simulink model "DynamicModel_Cascaded_BAv02"  (R2022b)
settings: Solver=VariableStepAuto  StartTime=0.0  StopTime=9*3600  MaxStep=0.2  RelTol=1e-3
undefined symbols (not defined in the file): driver, getPhysicalConstants, param, route, weatherSim
libraries: slpidlib x4
settings Model: NumberOfSteps=100  Creator=giaco  LastModifiedBy=giaco

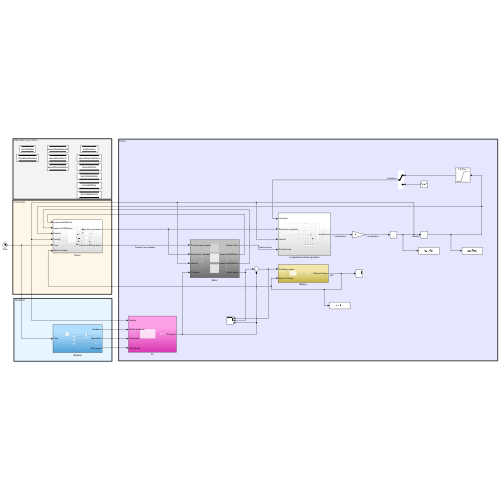
[thumbnail: Simulink's stored preview of the top-level diagram]
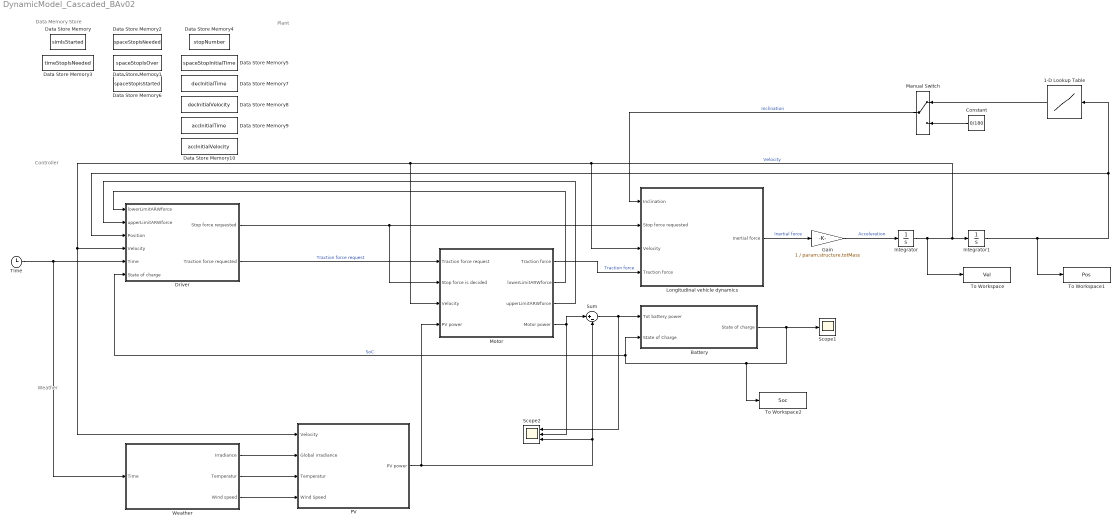
== system DynamicModel_Cascaded_BAv02 ==
  note: Weather
  note: Controller
  note: Plant
  note: Data Memory Store
  1-D Lookup Table : Lookup_n-D  NumberOfTableDimensions=1  BreakpointsForDimension1=route.dist(1:end-1)  Table=route.inclSmooth  InternalRulePriority=Speed  RndMeth=Simplest
  Battery : Subsystem
  Constant : Constant  Value=0/180
  Data Store Memory : DataStoreMemory  DataStoreName=simIsStarted  WriteAfterWriteMsg=warning  InitialValue=true  ShowAdditionalParam=off  OutDataTypeStr=boolean
  Data Store Memory1 : DataStoreMemory  DataStoreName=spaceStopIsOver  WriteAfterWriteMsg=warning  InitialValue=false  ShowAdditionalParam=off  OutDataTypeStr=boolean
  Data Store Memory10 : DataStoreMemory  DataStoreName=accInitialVelocity  WriteAfterWriteMsg=warning  VectorParams1D=off  ShowAdditionalParam=off  OutDataTypeStr=double
  Data Store Memory2 : DataStoreMemory  DataStoreName=spaceStopIsNeeded  WriteAfterWriteMsg=warning  InitialValue=false  ShowAdditionalParam=off  OutDataTypeStr=boolean
  Data Store Memory3 : DataStoreMemory  DataStoreName=timeStopIsNeeded  WriteAfterWriteMsg=warning  InitialValue=false  ShowAdditionalParam=off  OutDataTypeStr=boolean
  Data Store Memory4 : DataStoreMemory  DataStoreName=stopNumber  WriteAfterWriteMsg=warning  InitialValue=2  VectorParams1D=off  ShowAdditionalParam=off  OutDataTypeStr=int8
  Data Store Memory5 : DataStoreMemory  DataStoreName=spaceStopInitialTime  WriteAfterWriteMsg=warning  VectorParams1D=off  ShowAdditionalParam=off  OutDataTypeStr=double
  Data Store Memory6 : DataStoreMemory  DataStoreName=spaceStopIsStarted  WriteAfterWriteMsg=warning  InitialValue=false  ShowAdditionalParam=off  OutDataTypeStr=boolean
  Data Store Memory7 : DataStoreMemory  DataStoreName=decInitialTime  WriteAfterWriteMsg=warning  VectorParams1D=off  ShowAdditionalParam=off  OutDataTypeStr=double
  Data Store Memory8 : DataStoreMemory  DataStoreName=decInitialVelocity  WriteAfterWriteMsg=warning  VectorParams1D=off  ShowAdditionalParam=off  OutDataTypeStr=double
  Data Store Memory9 : DataStoreMemory  DataStoreName=accInitialTime  WriteAfterWriteMsg=warning  VectorParams1D=off  ShowAdditionalParam=off  OutDataTypeStr=double
  Driver : Subsystem
  Gain : Gain  Gain=1 / param.structure.totMass
  Integrator : Integrator
  Integrator1 : Integrator
  Longitudinal vehicle dynamics : Subsystem
  Manual Switch : ManualSwitch
  Motor : Subsystem
  PV : Subsystem
  Scope1 : Scope
  Scope2 : Scope  NumInputPorts=3
  Sum : Sum  Inputs=|+-
  Time : Clock
  To Workspace : ToWorkspace  VariableName=Vel  SaveFormat=Timeseries  SampleTime=-1
  To Workspace1 : ToWorkspace  VariableName=Pos  SaveFormat=Timeseries  SampleTime=-1
  To Workspace2 : ToWorkspace  VariableName=Soc  SaveFormat=Timeseries  SampleTime=-1
  Weather : Subsystem
  wires:
  Longitudinal vehicle dynamics/1(Inertial force) -> Gain/1  "Inertial force"
  Gain/1 -> Integrator/1  "Acceleration"
  Integrator/1 -> Integrator1/1, Longitudinal vehicle dynamics/3(Velocity), Motor/3(Velocity), PV/1(Velocity), Driver/4(Velocity), To Workspace/1  "Velocity"
  Motor/1(Traction force) -> Longitudinal vehicle dynamics/4(Traction force)  "Traction force"
  Integrator1/1 -> To Workspace1/1, 1-D Lookup Table/1, Driver/3(Position)
  1-D Lookup Table/1 -> Manual Switch/1
  Constant/1 -> Manual Switch/2
  Manual Switch/1 -> Longitudinal vehicle dynamics/1(Inclination)  "Inclination"
  Driver/2(Traction force requested) -> Motor/1(Traction force request)  "Traction force request"
  Sum/1 -> Scope2/1, Battery/1(Tot battery power)
  Motor/4(Motor power) -> Sum/1, Scope2/2
  PV/1(PV power) -> Sum/2, Scope2/3, Motor/4(PV power)
  Weather/1(Irradiance) -> PV/2(Global irradiance)
  Weather/2(Temperatur) -> PV/3(Temperatur)
  Weather/3(Wind speed) -> PV/4(Wind Speed)
  Battery/1(State of charge) -> To Workspace2/1, Battery/2(State of Charge), Driver/6(State of charge), Scope1/1  "SoC"
  Time/1 -> Weather/1(Time), Driver/5(Time)
  Driver/1(Stop force requested) -> Motor/2(Stop force is decided), Longitudinal vehicle dynamics/2(Stop force requested)
  Motor/2(lowerLimitARWforce) -> Driver/1(lowerLimitARWforce)
  Motor/3(upperLimitARWforce) -> Driver/2(upperLimitARWforce)

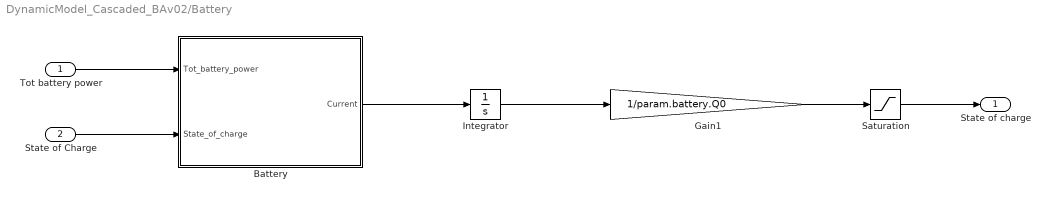
== system DynamicModel_Cascaded_BAv02/Battery ==
  Tot battery power : Inport
  State of Charge : Inport  Port=2
  Battery : MATLAB Function  TreatAsAtomicUnit=on
  Gain1 : Gain  Gain=1/param.battery.Q0
  Integrator : Integrator  InitialCondition=param.battery.Q0
  Saturation : Saturate  UpperLimit=1  LowerLimit=0
  State of charge : Outport
  wires:
  State of Charge/1 -> Battery/2(State_of_charge)
  Battery/1(Current) -> Integrator/1
  Integrator/1 -> Gain1/1
  Gain1/1 -> Saturation/1
  Tot battery power/1 -> Battery/1(Tot_battery_power)
  Saturation/1 -> State of charge/1

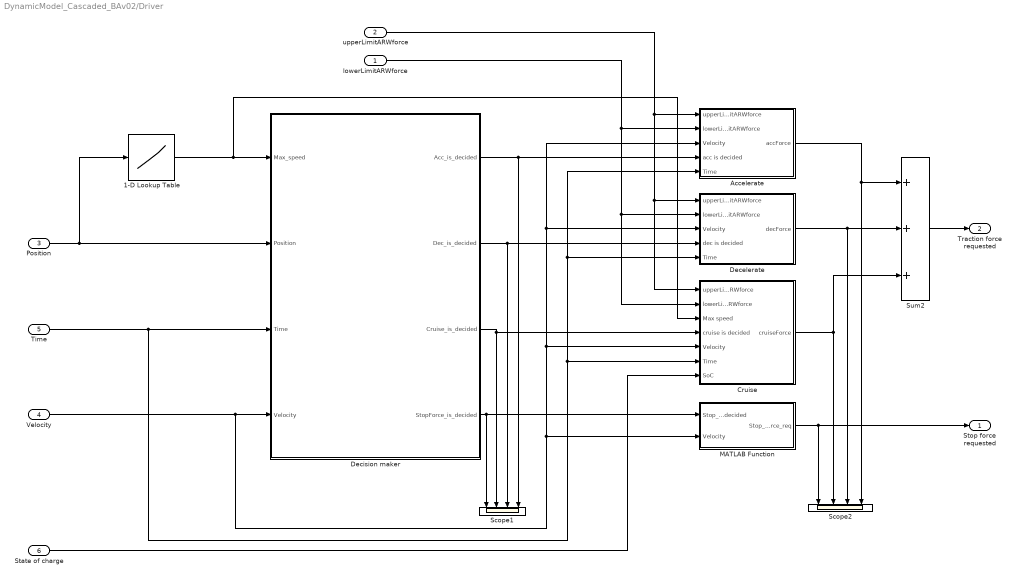
== system DynamicModel_Cascaded_BAv02/Driver ==
  lowerLimitARWforce : Inport
  upperLimitARWforce : Inport  Port=2
  Position : Inport  Port=3
  Velocity : Inport  Port=4
  Time : Inport  Port=5
  State of charge : Inport  Port=6
  1-D Lookup Table : Lookup_n-D  NumberOfTableDimensions=1  BreakpointsForDimension1=route.dist  Table=route.maxSpeed  InternalRulePriority=Speed  RndMeth=Simplest
  Accelerate : Subsystem
  Cruise : Subsystem
  Decelerate : Subsystem
  Decision maker : MATLAB Function  TreatAsAtomicUnit=on
  MATLAB Function : MATLAB Function  TreatAsAtomicUnit=on
  Scope1 : Scope  NumInputPorts=4
  Scope2 : Scope  NumInputPorts=4
  Sum2 : Sum  Inputs=+++
  Stop force requested : Outport
  Traction force requested : Outport  Port=2
  wires:
  1-D Lookup Table/1 -> Cruise/3(Max speed), Decision maker/1(Max_speed)
  Sum2/1 -> Traction force requested/1
  Decision maker/1(Acc_is_decided) -> Accelerate/4(acc is decided), Scope1/4
  Accelerate/1(accForce) -> Scope2/4, Sum2/1
  Decision maker/2(Dec_is_decided) -> Scope1/3, Decelerate/4(dec is decided)
  Decelerate/1(decForce) -> Scope2/3, Sum2/2
  Decision maker/3(Cruise_is_decided) -> Scope1/2, Cruise/4(cruise is decided)
  Cruise/1(cruiseForce) -> Scope2/2, Sum2/3
  MATLAB Function/1(Stop_force_req) -> Scope2/1, Stop force requested/1
  Decision maker/4(StopForce_is_decided) -> MATLAB Function/1(Stop_force_is_decided), Scope1/1
  upperLimitARWforce/1 -> Decelerate/1(upperLimitARWforce), Cruise/1(upperLimitARWforce), Accelerate/1(upperLimitARWforce)
  lowerLimitARWforce/1 -> Accelerate/2(lowerLimitARWforce), Decelerate/2(lowerLimitARWforce), Cruise/2(lowerLimitARWforce)
  Velocity/1 -> Accelerate/3(Velocity), Decelerate/3(Velocity), Cruise/5(Velocity), MATLAB Function/2(Velocity), Decision maker/4(Velocity)
  Time/1 -> Decision maker/3(Time), Cruise/6(Time), Accelerate/5(Time), Decelerate/5(Time)
  Position/1 -> 1-D Lookup Table/1, Decision maker/2(Position)
  State of charge/1 -> Cruise/7(SoC)

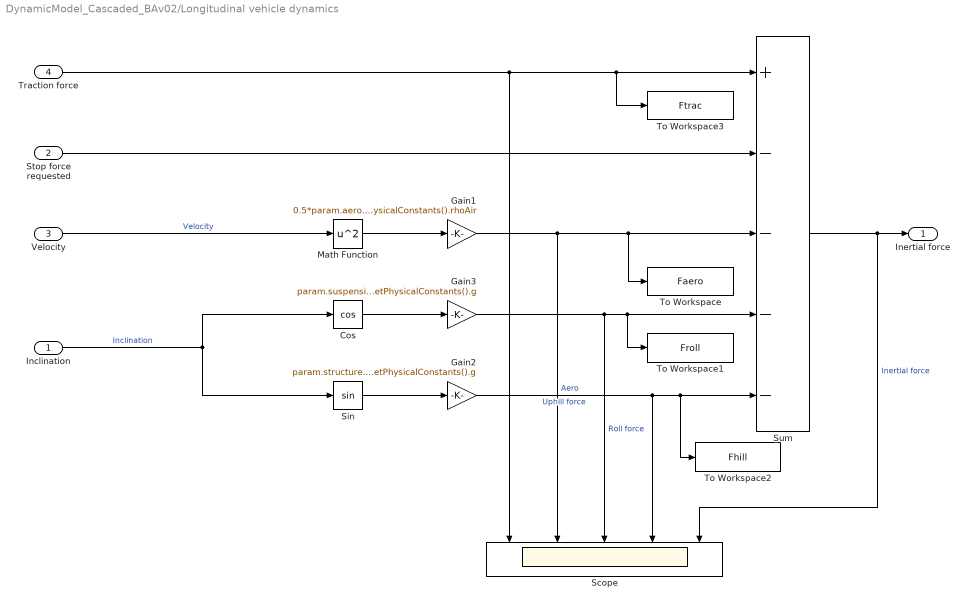
== system DynamicModel_Cascaded_BAv02/Longitudinal vehicle dynamics ==
  Inclination : Inport
  Stop force requested : Inport  Port=2
  Velocity : Inport  Port=3
  Traction force : Inport  Port=4
  Cos : Trigonometry  Operator=cos
  Gain1 : Gain  Gain=0.5*param.aero.AfCd*getPhysicalConstants().rhoAir
  Gain2 : Gain  Gain=param.structure.totMass*getPhysicalConstants().g
  Gain3 : Gain  Gain=param.suspension.cR*param.structure.totMass*getPhysicalConstants().g
  Math Function : Math  Operator=square
  Scope : Scope  NumInputPorts=5
  Sin : Trigonometry
  Sum : Sum  Inputs=+----
  To Workspace : ToWorkspace  VariableName=Faero  SaveFormat=Timeseries  SampleTime=-1
  To Workspace1 : ToWorkspace  VariableName=Froll  SaveFormat=Timeseries  SampleTime=-1
  To Workspace2 : ToWorkspace  VariableName=Fhill  SaveFormat=Timeseries  SampleTime=-1
  To Workspace3 : ToWorkspace  VariableName=Ftrac  SaveFormat=Timeseries  SampleTime=-1
  Inertial force : Outport
  wires:
  Traction force/1 -> To Workspace3/1, Sum/1, Scope/1
  Gain1/1 -> To Workspace/1, Sum/3, Scope/2  "Aero"
  Gain3/1 -> To Workspace1/1, Sum/4, Scope/3  "Roll force"
  Cos/1 -> Gain3/1
  Math Function/1 -> Gain1/1
  Inclination/1 -> Cos/1, Sin/1  "Inclination"
  Sin/1 -> Gain2/1
  Gain2/1 -> To Workspace2/1, Sum/5, Scope/4  "Uphill force"
  Velocity/1 -> Math Function/1  "Velocity"
  Sum/1 -> Inertial force/1, Scope/5  "Inertial force"
  Stop force requested/1 -> Sum/2

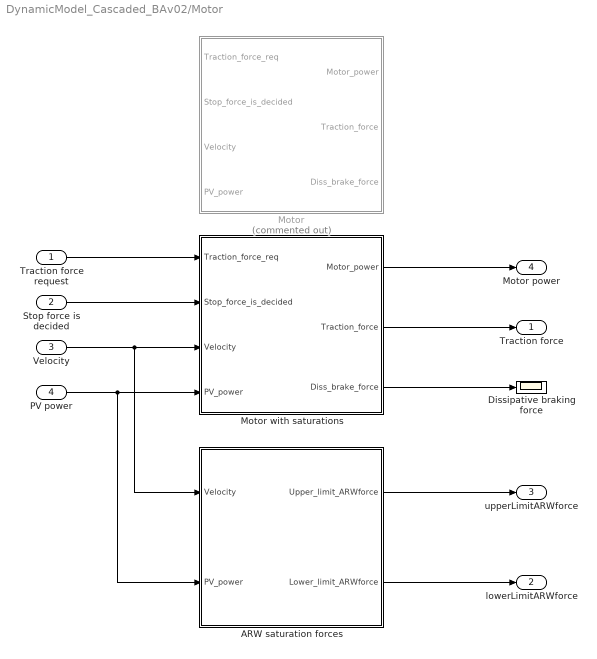
== system DynamicModel_Cascaded_BAv02/Motor ==
  Traction force request : Inport
  Stop force is decided : Inport  Port=2
  Velocity : Inport  Port=3
  PV power : Inport  Port=4
  ARW saturation forces : MATLAB Function  TreatAsAtomicUnit=on
  Dissipative braking force : Scope
  Motor : MATLAB Function  Commented=on  TreatAsAtomicUnit=on
  Motor with saturations : MATLAB Function  TreatAsAtomicUnit=on
  Traction force : Outport
  lowerLimitARWforce : Outport  Port=2
  upperLimitARWforce : Outport  Port=3
  Motor power : Outport  Port=4
  wires:
  Traction force request/1 -> Motor with saturations/1(Traction_force_req)
  Velocity/1 -> ARW saturation forces/1(Velocity), Motor with saturations/3(Velocity)
  Motor with saturations/1(Motor_power) -> Motor power/1
  Motor with saturations/2(Traction_force) -> Traction force/1
  Motor with saturations/3(Diss_brake_force) -> Dissipative braking force/1
  PV power/1 -> ARW saturation forces/2(PV_power), Motor with saturations/4(PV_power)
  Stop force is decided/1 -> Motor with saturations/2(Stop_force_is_decided)
  ARW saturation forces/1(Upper_limit_ARWforce) -> upperLimitARWforce/1
  ARW saturation forces/2(Lower_limit_ARWforce) -> lowerLimitARWforce/1

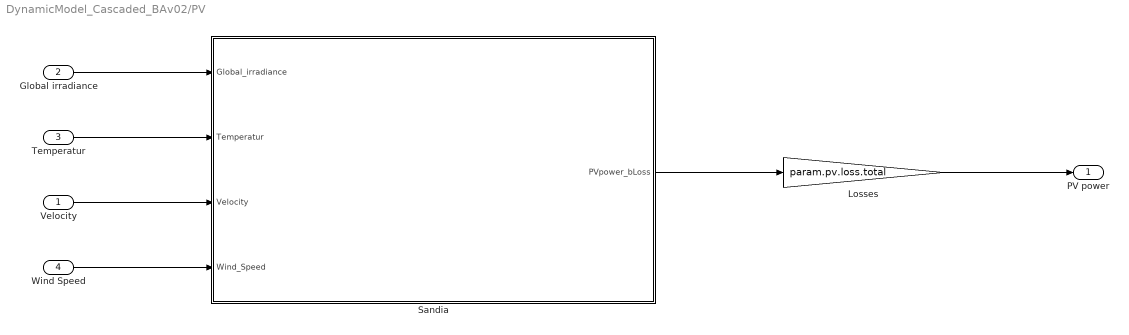
== system DynamicModel_Cascaded_BAv02/PV ==
  Velocity : Inport
  Global irradiance : Inport  Port=2
  Temperatur : Inport  Port=3
  Wind Speed : Inport  Port=4
  Losses : Gain  Gain=param.pv.loss.total
  Sandia : MATLAB Function  TreatAsAtomicUnit=on
  PV power : Outport
  wires:
  Global irradiance/1 -> Sandia/1(Global_irradiance)
  Temperatur/1 -> Sandia/2(Temperatur)
  Sandia/1(PVpower_bLoss) -> Losses/1
  Losses/1 -> PV power/1
  Velocity/1 -> Sandia/3(Velocity)
  Wind Speed/1 -> Sandia/4(Wind_Speed)

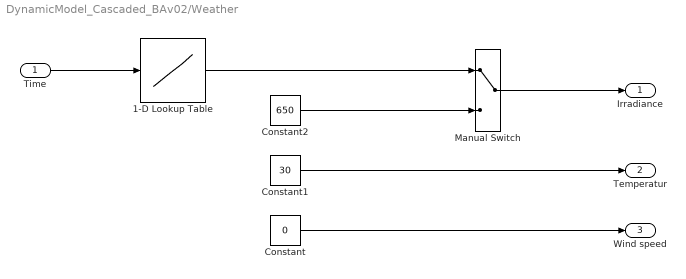
== system DynamicModel_Cascaded_BAv02/Weather ==
  Time : Inport
  1-D Lookup Table : Lookup_n-D  NumberOfTableDimensions=1  BreakpointsForDimension1=weatherSim.irradiance.timeSec  Table=weatherSim.irradiance.GtotalSec  InternalRulePriority=Speed  RndMeth=Simplest
  Constant : Constant  Value=0
  Constant1 : Constant  Value=30
  Constant2 : Constant  Value=650
  Manual Switch : ManualSwitch
  Irradiance : Outport
  Temperatur : Outport  Port=2
  Wind speed : Outport  Port=3
  wires:
  Constant1/1 -> Temperatur/1
  Constant2/1 -> Manual Switch/2
  Constant/1 -> Wind speed/1
  Manual Switch/1 -> Irradiance/1
  1-D Lookup Table/1 -> Manual Switch/1
  Time/1 -> 1-D Lookup Table/1

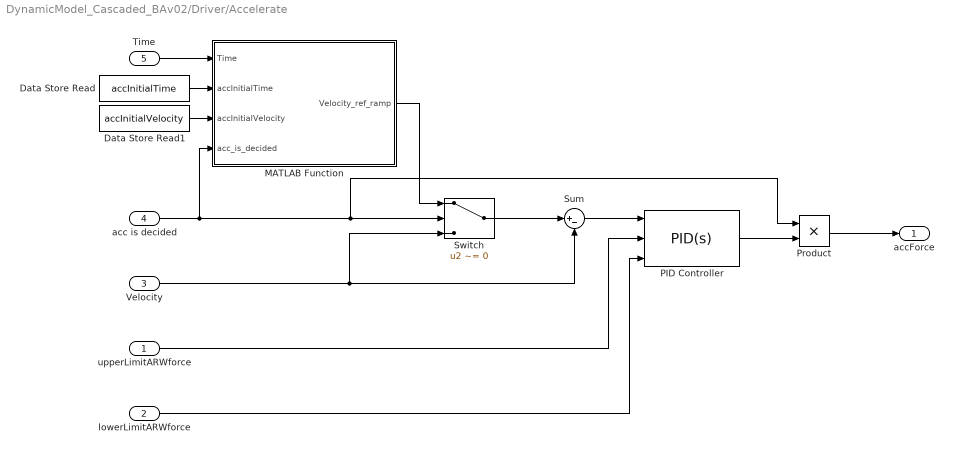
== system DynamicModel_Cascaded_BAv02/Driver/Accelerate ==
  upperLimitARWforce : Inport
  lowerLimitARWforce : Inport  Port=2
  Velocity : Inport  Port=3
  acc is decided : Inport  Port=4
  Time : Inport  Port=5
  Data Store Read : DataStoreRead  DataStoreName=accInitialTime  IndexOptions=Index vector (dialog)  Indices=1  OutputSizes=1
  Data Store Read1 : DataStoreRead  DataStoreName=accInitialVelocity  IndexOptions=Index vector (dialog)  Indices=1  OutputSizes=1
  MATLAB Function : MATLAB Function  TreatAsAtomicUnit=on
  PID Controller : slpidlib/PID Controller  Controller=PID  Form=Ideal  TimeDomain=Continuous-time  UseExternalTs=off  SampleTime=-1  IntegratorMethod=Forward Euler  FilterMethod=Forward Euler  ControllerParametersSource=internal  P=4000  I=1/1  UseKiTs=off  D=0  N=100  UseFilter=on  TunerSelectOption=Transfer Function Based (PID Tuner App)  InitialConditionSource=internal  InitialConditionForIntegrator=0  InitialConditionForFilter=0  DifferentiatorICPrevScaledInput=0  ExternalReset=none  TrackingMode=off  Kt=1  LimitOutput=on  SatLimitsSource=external  UpperSaturationLimit=param.motor.maxTorque * param.motor.transmissionRatio / param.suspension.rWheel  LowerSaturationLimit=param.motor.minTorque * param.motor.transmissionRatio / param.suspension.rWheel  LinearizeAsGain=on  AntiWindupMode=none  Kb=1  LimitIntegrator=off  UpperIntegratorSaturationLimit=inf  LowerIntegratorSaturationLimit=-inf  POutMin=[]  POutMax=[]  IOutMin=[]  IOutMax=[]  DOutMin=[]  DOutMax=[]  NOutMin=[]  NOutMax=[]  SumOutMin=[]  SumOutMax=[]  SaturationOutMin=[]  SaturationOutMax=[]  PParamMin=[]  PParamMax=[]  IParamMin=[]  IParamMax=[]  DParamMin=[]  DParamMax=[]  NParamMin=[]  NParamMax=[]  KbParamMin=[]  KbParamMax=[]  KtParamMin=[]  KtParamMax=[]  KbOutMin=[]  KbOutMax=[]  KtOutMin=[]  KtOutMax=[]  IntegratorOutMin=[]  IntegratorOutMax=[]  FilterOutMin=[]  FilterOutMax=[]  SumI1OutMin=[]  SumI1OutMax=[]  SumI2OutMin=[]  SumI2OutMax=[]  SumI3OutMin=[]  SumI3OutMax=[]  SumI4OutMin=[]  SumI4OutMax=[]  SumDOutMin=[]  SumDOutMax=[]  DifferentiatorOutMin=[]  DifferentiatorOutMax=[]  FilterDiffOutCoefMin=[]  FilterDiffOutCoefMax=[]  ReciprocalOutMin=[]  ReciprocalOutMax=[]  SumDenOutMin=[]  SumDenOutMax=[]  SumNumOutMin=[]  SumNumOutMax=[]  DivideOutMin=[]  DivideOutMax=[]  UdiffTsProdOutMin=[]  UdiffTsProdOutMax=[]  NTsProdOutMin=[]  NTsProdOutMax=[]  UintegralTsProdOutMin=[]  UintegralTsProdOutMax=[]  UngainTsProdOutMin=[]  UngainTsProdOutMax=[]  ClampingZeroOutDataTypeStr=Inherit: Inherit via back propagation  ClampingZeroOutMin=[]  ClampingZeroOutMax=[]  FilterDenConstantOutDataTypeStr=Inherit: Inherit via back propagation  FilterDenConstantOutMin=[]  FilterDenConstantOutMax=[]  PCopyOutDataTypeStr=Inherit: Inherit via back propagation  PCopyOutMin=[]  PCopyOutMax=[]  NCopyOutDataTypeStr=Inherit: Inherit via back propagation  NCopyOutMin=[]  NCopyOutMax=[]  IntegratorContinuousStateAttributes=''  IntegratorStateMustResolveToSignalObject=off  IntegratorRTWStateStorageClass=Auto  FilterContinuousStateAttributes=''  FilterStateMustResolveToSignalObject=off  FilterRTWStateStorageClass=Auto  ParallelPVariant=Passthrough  IdealPVariant=InternalParameters  IVariant=InternalParameters  DVariant=InternalParameters  IntegratorVariant=Continuous  SatVariant=External  AWVariant=Passthrough  PCopyVariant=Disabled  TRVariant=Disabled  FdbkBlocksVariant=Forward  IdealPFdbkVariant=Disabled  SatFdbkVariant=Disabled  DerivativeFilterVariant=ContFilter  NVariant=InternalParameters  NCopyVariant=Disabled  FilterICVariant=InternalICsFilter  IntegratorICVariant=InternalICs  ExternalResetVariant=Disabled  TRSumVariant=Passthrough  SumFdbkVariant=Disabled  SumVariant=Sum_PID  TsampFilterVariant=InternalTs  TsampNgainVariant=Passthrough  TsampIntegralVariant=Passthrough  ExternalSaturationOutDataTypeStr=Inherit: Same as second input
  Product : Product
  Sum : Sum  Inputs=|+-
  Switch : Switch  Criteria=u2 ~= 0  SaturateOnIntegerOverflow=off  InputSameDT=off
  accForce : Outport
  wires:
  acc is decided/1 -> MATLAB Function/4(acc_is_decided), Product/1, Switch/2
  Switch/1 -> Sum/1
  Velocity/1 -> Sum/2, Switch/3
  Sum/1 -> PID Controller/1
  PID Controller/1 -> Product/2
  Product/1 -> accForce/1
  Time/1 -> MATLAB Function/1(Time)
  MATLAB Function/1(Velocity_ref_ramp) -> Switch/1
  Data Store Read/1 -> MATLAB Function/2(accInitialTime)
  Data Store Read1/1 -> MATLAB Function/3(accInitialVelocity)
  upperLimitARWforce/1 -> PID Controller/2
  lowerLimitARWforce/1 -> PID Controller/3

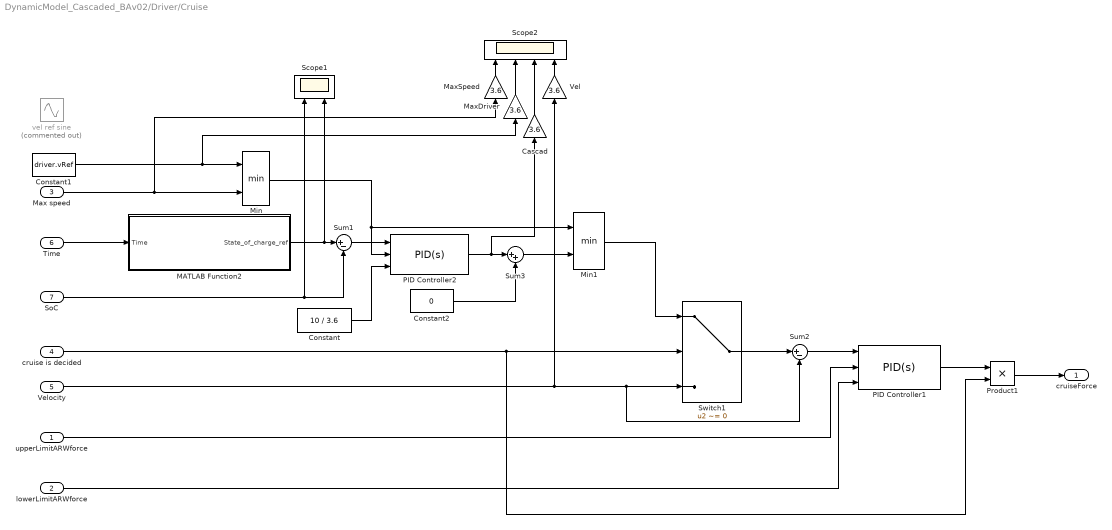
== system DynamicModel_Cascaded_BAv02/Driver/Cruise ==
  upperLimitARWforce : Inport
  lowerLimitARWforce : Inport  Port=2
  Max speed : Inport  Port=3
  cruise is decided : Inport  Port=4
  Velocity : Inport  Port=5
  Time : Inport  Port=6
  SoC : Inport  Port=7
  Cascad : Gain  Gain=3.6
  Constant : Constant  Value=10 / 3.6
  Constant1 : Constant  Value=driver.vRef
  Constant2 : Constant  Value=0
  MATLAB Function2 : MATLAB Function  TreatAsAtomicUnit=on
  MaxDriver : Gain  Gain=3.6
  MaxSpeed : Gain  Gain=3.6
  Min : MinMax  Inputs=2
  Min1 : MinMax  Inputs=2
  PID Controller1 : slpidlib/PID Controller  Controller=PID  Form=Parallel  TimeDomain=Continuous-time  UseExternalTs=off  SampleTime=-1  IntegratorMethod=Forward Euler  FilterMethod=Forward Euler  ControllerParametersSource=internal  P=80  I=1  UseKiTs=off  D=0  N=100  UseFilter=on  TunerSelectOption=Transfer Function Based (PID Tuner App)  InitialConditionSource=internal  InitialConditionForIntegrator=0  InitialConditionForFilter=0  DifferentiatorICPrevScaledInput=0  ExternalReset=none  TrackingMode=off  Kt=1  LimitOutput=on  SatLimitsSource=external  UpperSaturationLimit=param.motor.maxTorque * param.motor.transmissionRatio / param.suspension.rWheel  LowerSaturationLimit=param.motor.minTorque * param.motor.transmissionRatio / param.suspension.rWheel  LinearizeAsGain=on  AntiWindupMode=none  Kb=1  LimitIntegrator=off  UpperIntegratorSaturationLimit=inf  LowerIntegratorSaturationLimit=-inf  POutMin=[]  POutMax=[]  IOutMin=[]  IOutMax=[]  DOutMin=[]  DOutMax=[]  NOutMin=[]  NOutMax=[]  SumOutMin=[]  SumOutMax=[]  SaturationOutMin=[]  SaturationOutMax=[]  PParamMin=[]  PParamMax=[]  IParamMin=[]  IParamMax=[]  DParamMin=[]  DParamMax=[]  NParamMin=[]  NParamMax=[]  KbParamMin=[]  KbParamMax=[]  KtParamMin=[]  KtParamMax=[]  KbOutMin=[]  KbOutMax=[]  KtOutMin=[]  KtOutMax=[]  IntegratorOutMin=[]  IntegratorOutMax=[]  FilterOutMin=[]  FilterOutMax=[]  SumI1OutMin=[]  SumI1OutMax=[]  SumI2OutMin=[]  SumI2OutMax=[]  SumI3OutMin=[]  SumI3OutMax=[]  SumI4OutMin=[]  SumI4OutMax=[]  SumDOutMin=[]  SumDOutMax=[]  DifferentiatorOutMin=[]  DifferentiatorOutMax=[]  FilterDiffOutCoefMin=[]  FilterDiffOutCoefMax=[]  ReciprocalOutMin=[]  ReciprocalOutMax=[]  SumDenOutMin=[]  SumDenOutMax=[]  SumNumOutMin=[]  SumNumOutMax=[]  DivideOutMin=[]  DivideOutMax=[]  UdiffTsProdOutMin=[]  UdiffTsProdOutMax=[]  NTsProdOutMin=[]  NTsProdOutMax=[]  UintegralTsProdOutMin=[]  UintegralTsProdOutMax=[]  UngainTsProdOutMin=[]  UngainTsProdOutMax=[]  ClampingZeroOutDataTypeStr=Inherit: Inherit via back propagation  ClampingZeroOutMin=[]  ClampingZeroOutMax=[]  FilterDenConstantOutDataTypeStr=Inherit: Inherit via back propagation  FilterDenConstantOutMin=[]  FilterDenConstantOutMax=[]  PCopyOutDataTypeStr=Inherit: Inherit via back propagation  PCopyOutMin=[]  PCopyOutMax=[]  NCopyOutDataTypeStr=Inherit: Inherit via back propagation  NCopyOutMin=[]  NCopyOutMax=[]  IntegratorContinuousStateAttributes=''  IntegratorStateMustResolveToSignalObject=off  IntegratorRTWStateStorageClass=Auto  FilterContinuousStateAttributes=''  FilterStateMustResolveToSignalObject=off  FilterRTWStateStorageClass=Auto  ParallelPVariant=InternalParameters  IdealPVariant=Disabled  IVariant=InternalParameters  DVariant=InternalParameters  IntegratorVariant=Continuous  SatVariant=External  AWVariant=Passthrough  PCopyVariant=Disabled  TRVariant=Disabled  FdbkBlocksVariant=Forward  IdealPFdbkVariant=Disabled  SatFdbkVariant=Disabled  DerivativeFilterVariant=ContFilter  NVariant=InternalParameters  NCopyVariant=Disabled  FilterICVariant=InternalICsFilter  IntegratorICVariant=InternalICs  ExternalResetVariant=Disabled  TRSumVariant=Passthrough  SumFdbkVariant=Disabled  SumVariant=Sum_PID  TsampFilterVariant=InternalTs  TsampNgainVariant=Passthrough  TsampIntegralVariant=Passthrough  ExternalSaturationOutDataTypeStr=Inherit: Same as second input
  PID Controller2 : slpidlib/PID Controller  Controller=PID  Form=Ideal  TimeDomain=Continuous-time  UseExternalTs=off  SampleTime=-1  IntegratorMethod=Forward Euler  FilterMethod=Forward Euler  ControllerParametersSource=internal  P=-500  I=1/600  UseKiTs=off  D=0  N=100  UseFilter=on  TunerSelectOption=Transfer Function Based (PID Tuner App)  InitialConditionSource=internal  InitialConditionForIntegrator=0  InitialConditionForFilter=0  DifferentiatorICPrevScaledInput=0  ExternalReset=none  TrackingMode=off  Kt=1  LimitOutput=on  SatLimitsSource=external  UpperSaturationLimit=inf  LowerSaturationLimit=-driver.vRef*0.9  LinearizeAsGain=on  AntiWindupMode=none  Kb=1  LimitIntegrator=off  UpperIntegratorSaturationLimit=inf  LowerIntegratorSaturationLimit=-inf  POutMin=[]  POutMax=[]  IOutMin=[]  IOutMax=[]  DOutMin=[]  DOutMax=[]  NOutMin=[]  NOutMax=[]  SumOutMin=[]  SumOutMax=[]  SaturationOutMin=[]  SaturationOutMax=[]  PParamMin=[]  PParamMax=[]  IParamMin=[]  IParamMax=[]  DParamMin=[]  DParamMax=[]  NParamMin=[]  NParamMax=[]  KbParamMin=[]  KbParamMax=[]  KtParamMin=[]  KtParamMax=[]  KbOutMin=[]  KbOutMax=[]  KtOutMin=[]  KtOutMax=[]  IntegratorOutMin=[]  IntegratorOutMax=[]  FilterOutMin=[]  FilterOutMax=[]  SumI1OutMin=[]  SumI1OutMax=[]  SumI2OutMin=[]  SumI2OutMax=[]  SumI3OutMin=[]  SumI3OutMax=[]  SumI4OutMin=[]  SumI4OutMax=[]  SumDOutMin=[]  SumDOutMax=[]  DifferentiatorOutMin=[]  DifferentiatorOutMax=[]  FilterDiffOutCoefMin=[]  FilterDiffOutCoefMax=[]  ReciprocalOutMin=[]  ReciprocalOutMax=[]  SumDenOutMin=[]  SumDenOutMax=[]  SumNumOutMin=[]  SumNumOutMax=[]  DivideOutMin=[]  DivideOutMax=[]  UdiffTsProdOutMin=[]  UdiffTsProdOutMax=[]  NTsProdOutMin=[]  NTsProdOutMax=[]  UintegralTsProdOutMin=[]  UintegralTsProdOutMax=[]  UngainTsProdOutMin=[]  UngainTsProdOutMax=[]  ClampingZeroOutDataTypeStr=Inherit: Inherit via back propagation  ClampingZeroOutMin=[]  ClampingZeroOutMax=[]  FilterDenConstantOutDataTypeStr=Inherit: Inherit via back propagation  FilterDenConstantOutMin=[]  FilterDenConstantOutMax=[]  PCopyOutDataTypeStr=Inherit: Inherit via back propagation  PCopyOutMin=[]  PCopyOutMax=[]  NCopyOutDataTypeStr=Inherit: Inherit via back propagation  NCopyOutMin=[]  NCopyOutMax=[]  IntegratorContinuousStateAttributes=''  IntegratorStateMustResolveToSignalObject=off  IntegratorRTWStateStorageClass=Auto  FilterContinuousStateAttributes=''  FilterStateMustResolveToSignalObject=off  FilterRTWStateStorageClass=Auto  ParallelPVariant=Passthrough  IdealPVariant=InternalParameters  IVariant=InternalParameters  DVariant=InternalParameters  IntegratorVariant=Continuous  SatVariant=External  AWVariant=Passthrough  PCopyVariant=Disabled  TRVariant=Disabled  FdbkBlocksVariant=Forward  IdealPFdbkVariant=Disabled  SatFdbkVariant=Disabled  DerivativeFilterVariant=ContFilter  NVariant=InternalParameters  NCopyVariant=Disabled  FilterICVariant=InternalICsFilter  IntegratorICVariant=InternalICs  ExternalResetVariant=Disabled  TRSumVariant=Passthrough  SumFdbkVariant=Disabled  SumVariant=Sum_PID  TsampFilterVariant=InternalTs  TsampNgainVariant=Passthrough  TsampIntegralVariant=Passthrough  ExternalSaturationOutDataTypeStr=Inherit: Same as second input
  Product1 : Product
  Scope1 : Scope  NumInputPorts=2
  Scope2 : Scope  NumInputPorts=4
  Sum1 : Sum  Inputs=|+-
  Sum2 : Sum  Inputs=|+-
  Sum3 : Sum  Inputs=|++
  Switch1 : Switch  Criteria=u2 ~= 0  SaturateOnIntegerOverflow=off  InputSameDT=off
  Vel : Gain  Gain=3.6
  vel ref sine : Sin  Commented=on  Amplitude=5  Bias=20  Frequency=1/120  SampleTime=0
  cruiseForce : Outport
  wires:
  Max speed/1 -> MaxSpeed/1, Min/2
  lowerLimitARWforce/1 -> PID Controller1/3
  upperLimitARWforce/1 -> PID Controller1/2
  PID Controller2/1 -> Cascad/1, Sum3/1
  Sum3/1 -> Min1/2
  Sum1/1 -> PID Controller2/1
  Min1/1 -> Switch1/1
  Sum2/1 -> PID Controller1/1
  SoC/1 -> Sum1/2, Scope1/1
  Constant2/1 -> Sum3/2
  MATLAB Function2/1(State_of_charge_ref) -> Scope1/2, Sum1/1
  Time/1 -> MATLAB Function2/1(Time)
  Product1/1 -> cruiseForce/1
  cruise is decided/1 -> Product1/2, Switch1/2
  PID Controller1/1 -> Product1/1
  Switch1/1 -> Sum2/1
  Velocity/1 -> Vel/1, Sum2/2, Switch1/3
  Constant/1 -> PID Controller2/3
  Constant1/1 -> MaxDriver/1, Min/1
  Min/1 -> Min1/1, PID Controller2/2
  Vel/1 -> Scope2/4
  Cascad/1 -> Scope2/3
  MaxSpeed/1 -> Scope2/1
  MaxDriver/1 -> Scope2/2

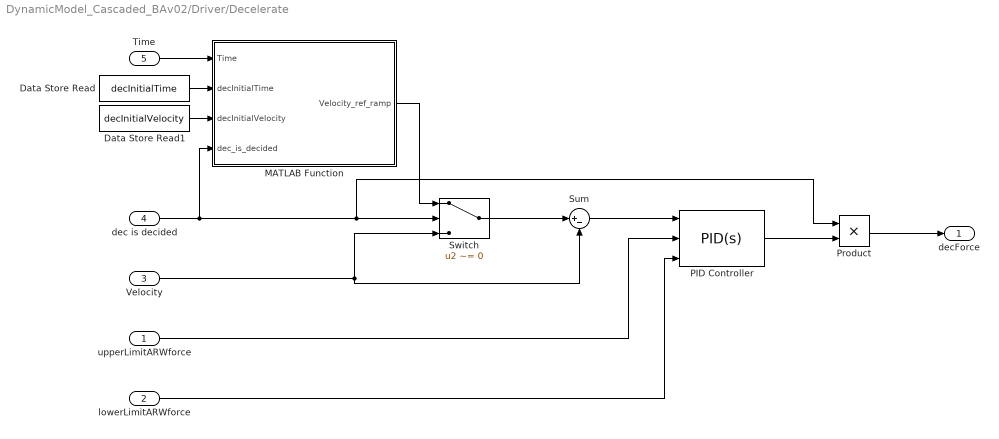
== system DynamicModel_Cascaded_BAv02/Driver/Decelerate ==
  upperLimitARWforce : Inport
  lowerLimitARWforce : Inport  Port=2
  Velocity : Inport  Port=3
  dec is decided : Inport  Port=4
  Time : Inport  Port=5
  Data Store Read : DataStoreRead  DataStoreName=decInitialTime  IndexOptions=Index vector (dialog)  Indices=1  OutputSizes=1
  Data Store Read1 : DataStoreRead  DataStoreName=decInitialVelocity  IndexOptions=Index vector (dialog)  Indices=1  OutputSizes=1
  MATLAB Function : MATLAB Function  TreatAsAtomicUnit=on
  PID Controller : slpidlib/PID Controller  Controller=PID  Form=Ideal  TimeDomain=Continuous-time  UseExternalTs=off  SampleTime=-1  IntegratorMethod=Forward Euler  FilterMethod=Forward Euler  ControllerParametersSource=internal  P=4000  I=1/1  UseKiTs=off  D=0  N=100  UseFilter=on  TunerSelectOption=Transfer Function Based (PID Tuner App)  InitialConditionSource=internal  InitialConditionForIntegrator=0  InitialConditionForFilter=0  DifferentiatorICPrevScaledInput=0  ExternalReset=none  TrackingMode=off  Kt=1  LimitOutput=on  SatLimitsSource=external  UpperSaturationLimit=param.motor.maxTorque * param.motor.transmissionRatio / param.suspension.rWheel  LowerSaturationLimit=param.motor.minTorque * param.motor.transmissionRatio / param.suspension.rWheel  LinearizeAsGain=on  AntiWindupMode=none  Kb=1  LimitIntegrator=off  UpperIntegratorSaturationLimit=inf  LowerIntegratorSaturationLimit=-inf  POutMin=[]  POutMax=[]  IOutMin=[]  IOutMax=[]  DOutMin=[]  DOutMax=[]  NOutMin=[]  NOutMax=[]  SumOutMin=[]  SumOutMax=[]  SaturationOutMin=[]  SaturationOutMax=[]  PParamMin=[]  PParamMax=[]  IParamMin=[]  IParamMax=[]  DParamMin=[]  DParamMax=[]  NParamMin=[]  NParamMax=[]  KbParamMin=[]  KbParamMax=[]  KtParamMin=[]  KtParamMax=[]  KbOutMin=[]  KbOutMax=[]  KtOutMin=[]  KtOutMax=[]  IntegratorOutMin=[]  IntegratorOutMax=[]  FilterOutMin=[]  FilterOutMax=[]  SumI1OutMin=[]  SumI1OutMax=[]  SumI2OutMin=[]  SumI2OutMax=[]  SumI3OutMin=[]  SumI3OutMax=[]  SumI4OutMin=[]  SumI4OutMax=[]  SumDOutMin=[]  SumDOutMax=[]  DifferentiatorOutMin=[]  DifferentiatorOutMax=[]  FilterDiffOutCoefMin=[]  FilterDiffOutCoefMax=[]  ReciprocalOutMin=[]  ReciprocalOutMax=[]  SumDenOutMin=[]  SumDenOutMax=[]  SumNumOutMin=[]  SumNumOutMax=[]  DivideOutMin=[]  DivideOutMax=[]  UdiffTsProdOutMin=[]  UdiffTsProdOutMax=[]  NTsProdOutMin=[]  NTsProdOutMax=[]  UintegralTsProdOutMin=[]  UintegralTsProdOutMax=[]  UngainTsProdOutMin=[]  UngainTsProdOutMax=[]  ClampingZeroOutDataTypeStr=Inherit: Inherit via back propagation  ClampingZeroOutMin=[]  ClampingZeroOutMax=[]  FilterDenConstantOutDataTypeStr=Inherit: Inherit via back propagation  FilterDenConstantOutMin=[]  FilterDenConstantOutMax=[]  PCopyOutDataTypeStr=Inherit: Inherit via back propagation  PCopyOutMin=[]  PCopyOutMax=[]  NCopyOutDataTypeStr=Inherit: Inherit via back propagation  NCopyOutMin=[]  NCopyOutMax=[]  IntegratorContinuousStateAttributes=''  IntegratorStateMustResolveToSignalObject=off  IntegratorRTWStateStorageClass=Auto  FilterContinuousStateAttributes=''  FilterStateMustResolveToSignalObject=off  FilterRTWStateStorageClass=Auto  ParallelPVariant=Passthrough  IdealPVariant=InternalParameters  IVariant=InternalParameters  DVariant=InternalParameters  IntegratorVariant=Continuous  SatVariant=External  AWVariant=Passthrough  PCopyVariant=Disabled  TRVariant=Disabled  FdbkBlocksVariant=Forward  IdealPFdbkVariant=Disabled  SatFdbkVariant=Disabled  DerivativeFilterVariant=ContFilter  NVariant=InternalParameters  NCopyVariant=Disabled  FilterICVariant=InternalICsFilter  IntegratorICVariant=InternalICs  ExternalResetVariant=Disabled  TRSumVariant=Passthrough  SumFdbkVariant=Disabled  SumVariant=Sum_PID  TsampFilterVariant=InternalTs  TsampNgainVariant=Passthrough  TsampIntegralVariant=Passthrough  ExternalSaturationOutDataTypeStr=Inherit: Same as second input
  Product : Product
  Sum : Sum  Inputs=|+-
  Switch : Switch  Criteria=u2 ~= 0  SaturateOnIntegerOverflow=off  InputSameDT=off
  decForce : Outport
  wires:
  dec is decided/1 -> MATLAB Function/4(dec_is_decided), Product/1, Switch/2
  Switch/1 -> Sum/1
  Velocity/1 -> Sum/2, Switch/3
  PID Controller/1 -> Product/2
  Sum/1 -> PID Controller/1
  Product/1 -> decForce/1
  Time/1 -> MATLAB Function/1(Time)
  Data Store Read1/1 -> MATLAB Function/3(decInitialVelocity)
  MATLAB Function/1(Velocity_ref_ramp) -> Switch/1
  Data Store Read/1 -> MATLAB Function/2(decInitialTime)
  upperLimitARWforce/1 -> PID Controller/2
  lowerLimitARWforce/1 -> PID Controller/3

== matlab function DynamicModel_Cascaded_BAv02/Motor/Motor ==
  data: Traction_force_req input; Stop_force_is_decided input; Velocity input; PV_power input; param parameter; Motor_power output; Traction_force output; Diss_brake_force output
function [Motor_power, Traction_force, Diss_brake_force] = Motor(Traction_force_req, Stop_force_is_decided, Velocity, PV_power, param)

Diss_brake_force = 0; %normally

maxElPowerMotBat = param.battery.maxPowerDelta .* param.battery.totNum + PV_power;
%Willans model
if maxElPowerMotBat >= 0
    maxMechPowerMotBat = maxElPowerMotBat * param.motor.efficiency - param.motor.p0;
else
    maxMechPowerMotBat = maxElPowerMotBat / param.motor.efficiency - param.motor.p0;
end % if

if Stop_force_is_decided
    Traction_force = 0;
    Motor_power = 0;

%condition for starting the simulation - avoid division with zero
elseif Velocity == 0
    Motor_power = param.motor.maxPower ./ 5;
    Traction_force = Traction_force_req ./ 5;
else
    
    %% POWER
    %conversion to torque
    tractionTorque = param.suspension.rWheel/param.motor.transmissionRatio .* Traction_force_req;
    %limits on the torque
    tractionTorque = min(tractionTorque, param.motor.maxTorque);
    tractionTorque = max(tractionTorque, param.motor.minTorque);
    
    %conversion to angular velocity
    omega = param.motor.transmissionRatio/param.suspension.rWheel .* Velocity;
    
    
    %mechanical power
    mechPower = omega .* tractionTorque;
    %limits on the power
    mechPower = min(mechPower, maxMechPowerMotBat); %upper limit battery
%     minPowerMotBat = param.battery.minPower .* param.battery.totNum + PV_power;
%     mechPower = max(mechPower, minPowerMotBat); %lower limit battery

    mechPower = min(mechPower, param.motor.maxPower); %upper limit motor
    mechPower = max(mechPower, param.motor.minPower); %lower limit motor
    
    
    %electrical power / motor power
    if mechPower >= 0
        Motor_power = (mechPower + param.motor.p0) / param.motor.efficiency;
    else
        Motor_power = (mechPower + param.motor.p0) * param.motor.efficiency;
    end % if

    %% FORCE
    Traction_force = mechPower ./ Velocity;

    %additional dissapitive braking force
    deltaBrake = Traction_force_req - Traction_force;
    if deltaBrake < 0
        Diss_brake_force = deltaBrake;
        Traction_force = Traction_force + Diss_brake_force;
    end %if
end % if

== matlab function DynamicModel_Cascaded_BAv02/Motor/Motor with saturations ==
  data: Traction_force_req input; Stop_force_is_decided input; Velocity input; PV_power input; param parameter; Motor_power output; Traction_force output; Diss_brake_force output
function [Motor_power, Traction_force, Diss_brake_force] = Motor(Traction_force_req, Stop_force_is_decided, Velocity, PV_power, param)

Diss_brake_force = 0;

maxElPowerMotBat = param.battery.maxPowerDelta .* param.battery.totNum + PV_power;
%Willans model
if maxElPowerMotBat >= 0
    maxMechPowerMotBat = maxElPowerMotBat * param.motor.efficiency - param.motor.p0;
else
    maxMechPowerMotBat = maxElPowerMotBat / param.motor.efficiency - param.motor.p0;
end % if

%% 
if Stop_force_is_decided
    Traction_force = 0;
    Motor_power = 0;

else
%% Conversions
    tractionTorqueReq = Traction_force_req * param.suspension.rWheel/param.motor.transmissionRatio;
    omegaMot = Velocity * param.motor.transmissionRatio/param.suspension.rWheel;

%% Limits
    tractionTorque = min(tractionTorqueReq, param.motor.maxTorque);
    tractionTorque = max(tractionTorque, param.motor.minTorque);
    tractionTorque = min(tractionTorque, maxMechPowerMotBat / max(omegaMot, 1e-8)); %upper limit power battery
    tractionTorque = min(tractionTorque, param.motor.maxPower / max(omegaMot, 1e-8)); %upper limit power motor
    tractionTorque = max(tractionTorque, param.motor.minPower / max(omegaMot, 1e-8)); %lower limit power motor    
    
%% Power
    mechPower = omegaMot * tractionTorque;
    %Willans model
    if mechPower >= 0
        Motor_power = (mechPower + param.motor.p0) / param.motor.efficiency;
    else
        Motor_power = (mechPower + param.motor.p0) * param.motor.efficiency;
    end % if

%% Force
    Traction_force = tractionTorque * param.motor.transmissionRatio / param.suspension.rWheel;

    %additional dissipative braking force
    deltaBrake = Traction_force_req - Traction_force;
    if deltaBrake < 0
        Diss_brake_force = deltaBrake;
        Traction_force = Traction_force + Diss_brake_force;
    end % if
end % if

== matlab function DynamicModel_Cascaded_BAv02/Motor/ARW saturation forces ==
  data: Velocity input; PV_power input; param parameter; Upper_limit_ARWforce output; Lower_limit_ARWforce output
function [Upper_limit_ARWforce, Lower_limit_ARWforce] = Motor(Velocity, PV_power, param)

maxElPowerMotBat = param.battery.maxPowerDelta .* param.battery.totNum + PV_power;
%Willans model
if maxElPowerMotBat >= 0
    maxMechPowerMotBat = maxElPowerMotBat * param.motor.efficiency - param.motor.p0;
else
    maxMechPowerMotBat = maxElPowerMotBat / param.motor.efficiency - param.motor.p0;
end % if

%% Lower limits
Lower_limit_ARWforce = max(param.motor.minTorque * param.motor.transmissionRatio/param.suspension.rWheel, param.motor.minPower / max(Velocity, 1e-8));

%% Upper limits
Upper_limit_ARWforce = min(param.motor.maxTorque * param.motor.transmissionRatio/param.suspension.rWheel, param.motor.maxPower / max(Velocity, 1e-8));
Upper_limit_ARWforce = min(Upper_limit_ARWforce, maxMechPowerMotBat / max(Velocity, 1e-8));

== matlab function DynamicModel_Cascaded_BAv02/Driver/Cruise/MATLAB Function2 ==
  data: Time input; State_of_charge_ref output; param parameter
function State_of_charge_ref = fcn(Time, param)

% State_of_charge_ref = 1 - 0.5 / (9*3600) * Time;
State_of_charge_ref = param.strategy.a*Time.^2 + param.strategy.b*Time + param.strategy.c;

== matlab function DynamicModel_Cascaded_BAv02/Driver/Accelerate/MATLAB Function ==
  data: Time input; Velocity_ref_ramp output; accInitialTime input; accInitialVelocity input; driver parameter; acc_is_decided input
function Velocity_ref_ramp = fcn(Time, accInitialTime, accInitialVelocity, driver, acc_is_decided)

Velocity_ref_ramp = 0;

if acc_is_decided
    Velocity_ref_ramp = driver.accRef .* (Time - accInitialTime) + accInitialVelocity;
end

== matlab function DynamicModel_Cascaded_BAv02/PV/Sandia ==
  data: Global_irradiance input; Temperatur input; Velocity input; PVpower_bLoss output; Wind_Speed input; param parameter
function PVpower_bLoss = fcn(Global_irradiance, Temperatur, Velocity, Wind_Speed, param)

type = "glass-cell-polymer";
mounting = "open rack";

relVelocity = Velocity - Wind_Speed;

switch type
    case "glass-cell-glass"
        if mounting == "open rack"
            a = -3.47;
            b = -0.0594;
            deltaTemp = 3;
        elseif mounting == "close roof mount"
            a = -2.98;
            b = -0.0471;
            deltaTemp = 1;
        end % if
    case "glass-cell-polymer"
        if mounting == "open rack"
            a = -3.56;
            b = -0.075;
            deltaTemp = 3;
        elseif mounting == "insulated back"
            a = -2.81;
            b = -0.0455;
            deltaTemp = 0;
        end % if
    case "polymer-thinfilm-steel"
        if mounting == "open rack"
            a = -3.58;
            b = -0.113;
            deltaTemp = 3;
        end % if
    otherwise
        a = -3.56;
        b = -0.075;
        deltaTemp = 3;
end % switch

tempModule = Global_irradiance.* exp(a + b.*relVelocity) + Temperatur;
tempCell = tempModule + Global_irradiance / param.pv.G0 * deltaTemp;


PVpower_bLoss = param.pv.area * Global_irradiance * param.pv.eff * (1 + param.pv.powerCoeff * (tempCell - param.pv.tempSTC));

== matlab function DynamicModel_Cascaded_BAv02/Battery/Battery ==
  data: Tot_battery_power input; State_of_charge input; Current output; param parameter
function Current = fcn(Tot_battery_power, State_of_charge, param)

%conversion to single battery power
Battery_power = Tot_battery_power ./ param.battery.totNum;

%OC parameters
Uoc = param.battery.k2 .* State_of_charge + param.battery.k1;
Ri = param.battery.k4 .* State_of_charge + param.battery.k3;

%solution of quadratic equation
Current = (Uoc - sqrt(Uoc^2 - 4*Battery_power*Ri)) / (2*Ri);

%Coulomb efficiency
Current = -1 * param.battery.effCoul .* Current;

== matlab function DynamicModel_Cascaded_BAv02/Driver/Decelerate/MATLAB Function ==
  data: Time input; Velocity_ref_ramp output; decInitialTime input; decInitialVelocity input; driver parameter; dec_is_decided input
function Velocity_ref_ramp = fcn(Time, decInitialTime, decInitialVelocity, driver, dec_is_decided)

Velocity_ref_ramp = 0;

if dec_is_decided
    Velocity_ref_ramp = driver.decRef .* (Time - decInitialTime) + decInitialVelocity;
end

== matlab function DynamicModel_Cascaded_BAv02/Driver/MATLAB Function ==
  data: Stop_force_is_decided input; Velocity input; Stop_force_req output
function Stop_force_req = fcn(Stop_force_is_decided, Velocity)

Stop_force_req = 0;

if Stop_force_is_decided
    Stop_force_req = 100 * sign(Velocity);
end % if

== matlab function DynamicModel_Cascaded_BAv02/Driver/Decision maker ==
  settings: updateMethod=DISCRETE
  data: Max_speed input; Position input; Time input; Velocity input; simIsStarted data_store_memory; spaceStopIsOver data_store_memory; timeStopIsNeeded data_store_memory; spaceStopIsNeeded data_store_memory; driver parameter; stopNumber data_store_memory; spaceStopIsStarted data_store_memory; Acc_is_decided output; Dec_is_decided output; Cruise_is_decided output; StopForce_is_decided output; spaceStopInitialTime data_store_memory; accInitialTime data_store_memory; accInitialVelocity data_store_memory; decInitialTime data_store_memory; decInitialVelocity data_store_memory
function [Acc_is_decided, Dec_is_decided, Cruise_is_decided, StopForce_is_decided] = decisionMaker(Max_speed, Position, Time, Velocity, driver)

global simIsStarted
global spaceStopIsOver
global timeStopIsNeeded;
global spaceStopIsNeeded;
global spaceStopIsStarted;

global stopNumber;
global spaceStopInitialTime;
global accInitialTime;
global accInitialVelocity;
global decInitialTime;
global decInitialVelocity;

Acc_is_decided = false;
Dec_is_decided = false;
Cruise_is_decided = false;
StopForce_is_decided = false;

controlVelocity = min(driver.vRef, Max_speed);

%% Check for stops
% Time stops assuming the simulation starts at 08.00 and ends at 17.00
stopTime = Time - Velocity ./ driver.decRef;

if ~timeStopIsNeeded && stopTime >= seconds(hours(8)+minutes(59)) %CHECK AGAINN %%%%%%%%%%%%%%%%%%%%%%%%%%%%%%%%%%%%%%%%
    timeStopIsNeeded = true;
    decInitialTime = Time; %initialization of time and velocity for ramp controller
    decInitialVelocity = Velocity;
end % if

% Space stops
stopDistance = Position - Velocity.^2 / (2 * driver.decRef);

if stopDistance >= driver.stopLocDist(stopNumber)
    spaceStopIsNeeded = true;
    decInitialTime = Time; %initialization of time and velocity for ramp controller
    decInitialVelocity = Velocity;
    stopNumber = stopNumber + 1;
end % if

%% Select control options

if simIsStarted || spaceStopIsOver                               % 1. Acceleration
    if  Velocity >= 0.9 * controlVelocity
        Cruise_is_decided = true;
        simIsStarted = false;
        spaceStopIsOver = false;
    else
        Acc_is_decided = true;
    end % if

    
elseif timeStopIsNeeded                                                 % 2. Deceleration
    if Velocity > driver.vRefStop
        Dec_is_decided = true;
    elseif Velocity <= driver.vRefStop
        StopForce_is_decided = true;
        Dec_is_decided = false;
    end % if

    
elseif spaceStopIsNeeded                                                % 2. Deceleration
    if spaceStopIsStarted
        spaceStopDuration = Time - spaceStopInitialTime;
        if spaceStopDuration >= 30*60
            spaceStopIsNeeded = false;
            spaceStopIsStarted = false;
            spaceStopIsOver = true;
            StopForce_is_decided = false;
            Acc_is_decided = true;
            accInitialTime = Time;
            accInitialVelocity = Velocity;
        else
            StopForce_is_decided = true;
            Acc_is_decided = false;
        end % if
    else
        if Velocity > driver.vRefStop
            Dec_is_decided = true;
        elseif Velocity <= driver.vRefStop
            spaceStopIsStarted = true;
            spaceStopInitialTime = Time;
            StopForce_is_decided = true;
            Dec_is_decided = false;
        end % if
    end % if


else                                                                        % 3. Cruise velocity
    Cruise_is_decided = true;
end % if
